simulink model "simple_model"  (R2013b)
settings: Solver=ode45  StartTime=0.0  StopTime=10.0  RelTol=1e-3
settings Model: Creator=Sander  LastModifiedBy=Sander

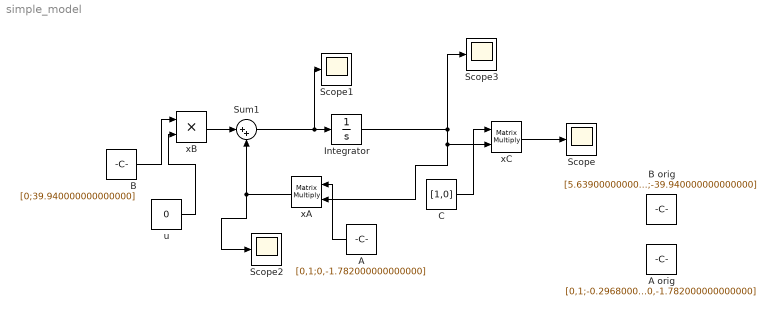
== system simple_model ==
  A : Constant  Value=[0,1;0,-1.782000000000000]  VectorParams1D=off
  A orig : Constant  Value=[0,1;-0.296800000000000,-1.782000000000000]  VectorParams1D=off
  B : Constant  Value=[0;39.940000000000000]  VectorParams1D=off
  B orig : Constant  Value=[5.639000000000000;-39.940000000000000]  VectorParams1D=off
  C : Constant  Value=[1,0]  VectorParams1D=off
  Integrator : Integrator  InitialCondition=[3;-2.8]
  Scope{,1..3} (4 alike) : Scope
      Scope1 settings: TimeRange=10  YMin=-10
      Scope2 settings: SaveName=ScopeData2
      Scope3 settings: SaveName=ScopeData3
  Sum1 : Sum  Inputs=|++
  u : Constant  Value=0  VectorParams1D=off
  xA : Product  Multiplication=Matrix(*)
  xB : Product
  xC : Product  Multiplication=Matrix(*)
  wires:
  B/1 -> xB/1
  A/1 -> xA/1
  xA/1 -> Scope2/1, Sum1/2
  xB/1 -> Sum1/1
  C/1 -> xC/1
  u/1 -> xB/2
  xC/1 -> Scope/1
  Integrator/1 -> Scope3/1, xA/2, xC/2
  Sum1/1 -> Scope1/1, Integrator/1
